simulink model "roadIntersection"  (R2017a)
settings: Solver=VariableStepAuto  StartTime=0  StopTime=40  MaxStep=0.05  RelTol=1e-3
model workspace (MAT data in the model file):
  GREEN_TIME = Simulink.Parameter
  GREEN_TIME.Value = 4
  GREEN_TIME.DataType = 'double'
  GREEN_TIME.Dimensions = [1 1]
  MIN_SAFE_DIST = Simulink.Parameter
  MIN_SAFE_DIST.Value = 1
  MIN_SAFE_DIST.DataType = 'double'
  MIN_SAFE_DIST.Dimensions = [1 1]
  PCROSS_TIME = Simulink.Parameter
  PCROSS_TIME.Value = 3
  PCROSS_TIME.DataType = 'double'
  PCROSS_TIME.Dimensions = [1 1]
  V_MIN = Simulink.Parameter
  V_MIN.Value = 0.25
  V_MIN.DataType = 'double'
  V_MIN.Dimensions = [1 1]
  V_TURN = Simulink.Parameter
  V_TURN.Value = 1.2
  V_TURN.DataType = 'double'
  V_TURN.Dimensions = [1 1]
  WORLD_SIZE = Simulink.Parameter
  WORLD_SIZE.Value = 8
  WORLD_SIZE.DataType = 'double'
  WORLD_SIZE.Dimensions = [1 1]
  YELLOW_TIME = Simulink.Parameter
  YELLOW_TIME.Value = 1
  YELLOW_TIME.DataType = 'double'
  YELLOW_TIME.Dimensions = [1 1]
  dt = Simulink.Parameter
  dt.Value = 0.05
  dt.DataType = 'double'
  dt.DocUnits = 'sec'
  dt.Dimensions = [1 1]
values from neighbouring files (symbols this model uses):
  D = getSimulinkBlockHandle('experiment/Orientation')    [configModel.m]
  m = rt.find('-isa','Simulink.BlockDiagram','-and','Name',mdl)    [configModel.m]
  MIN_SAFE_DIST = 1    [simulation.m]    (also in stateflowSim.m)
  V = getSimulinkBlockHandle('experiment/Velocity')    [configModel.m]
  WORLD_SIZE = 8    [simulation.m]    (also in stateflowSim.m)
  X = getSimulinkBlockHandle('experiment/Position')    [configModel.m]
undefined symbols (not defined in the file or in its folder): DrivingState, n, Stateflow
libraries: libraries x28
(part 1 of 2)
settings Model: Creator=larry  LastModifiedBy=larry
settings SolverCC: ZeroCrossControl=DisableAll  AutoInsertRateTranBlk=on

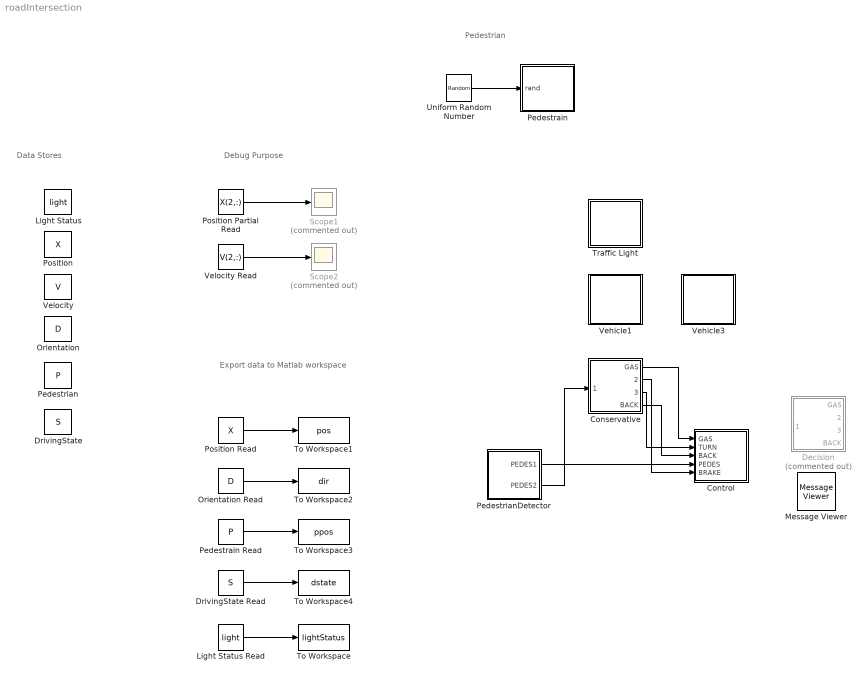
== system roadIntersection ==
  note: Data Stores
  note: Debug Purpose
  note: Export data to
      | Matlab workspace
  note: Pedestrian
  Conservative : Stateflow chart  TreatAsAtomicUnit=on
  Control : Stateflow chart  TreatAsAtomicUnit=on
  Decision : Stateflow chart  Commented=on  TreatAsAtomicUnit=on
  DrivingState : DataStoreMemory  DataStoreName=S  InitialValue=[DrivingState.Straight DrivingState.Straight DrivingState.Straight DrivingState.Straight]  ShowAdditionalParam=off  OutDataTypeStr=Enum: DrivingState
  DrivingState Read : DataStoreRead  DataStoreName=S
  Light Status : DataStoreMemory  DataStoreName=light  ShowAdditionalParam=off  OutDataTypeStr=double  Dimensions=1
  Light Status Read : DataStoreRead  DataStoreName=light
  Message Viewer : MessageViewer
  Orientation : DataStoreMemory  DataStoreName=D  InitialValue=[1 0 -1;0 1 0]  ShowAdditionalParam=off  OutDataTypeStr=double
  Orientation Read : DataStoreRead  DataStoreName=D
  Pedestrain : Stateflow chart  TreatAsAtomicUnit=on
  Pedestrain Read : DataStoreRead  DataStoreName=P
  Pedestrian : DataStoreMemory  DataStoreName=P  InitialValue=[-1; -1; -1; -1]  ShowAdditionalParam=off  OutDataTypeStr=double
  PedestrianDetector : Stateflow chart  TreatAsAtomicUnit=on
  Position : DataStoreMemory  DataStoreName=X  InitialValue=[-6 0.5 6;-0.5 4 0.5]  ShowAdditionalParam=off  OutDataTypeStr=double
  Position Read : DataStoreRead  DataStoreName=X
  Position Partial Read : DataStoreRead  DataStoreName=X  DataStoreElements=X(2,:)
  Scope1 : Scope  Commented=on
  Scope2 : Scope  Commented=on
  To Workspace : ToWorkspace  VariableName=lightStatus  SampleTime=-1
  To Workspace1 : ToWorkspace  VariableName=pos  SampleTime=-1
  To Workspace2 : ToWorkspace  VariableName=dir  SampleTime=-1
  To Workspace3 : ToWorkspace  VariableName=ppos  SampleTime=-1
  To Workspace4 : ToWorkspace  VariableName=dstate  SampleTime=-1
  Traffic Light : Stateflow chart  TreatAsAtomicUnit=on
  Uniform Random Number : UniformRandomNumber  Minimum=0  Maximum=5  SampleTime=0.05
  Vehicle1 : Stateflow chart  TreatAsAtomicUnit=on
  Vehicle3 : Stateflow chart  TreatAsAtomicUnit=on
  Velocity : DataStoreMemory  DataStoreName=V  InitialValue=[0 0 0;0 0 0]  ShowAdditionalParam=off  OutDataTypeStr=double
  Velocity Read : DataStoreRead  DataStoreName=V  DataStoreElements=V(2,:)
  wires:
  Light Status Read/1 -> To Workspace/1
  Position Partial Read/1 -> Scope1/1
  Velocity Read/1 -> Scope2/1
  Position Read/1 -> To Workspace1/1
  Orientation Read/1 -> To Workspace2/1
  Uniform Random Number/1 -> Pedestrain/1(rand)
  Pedestrain Read/1 -> To Workspace3/1
  Conservative/1(GAS) -> Control/1(GAS)
  Conservative/3(TURN) -> Control/2(TURN)
  Conservative/4(BACK) -> Control/3(BACK)
  PedestrianDetector/1(PEDES1) -> Control/4(PEDES)
  Conservative/2(BRAKE) -> Control/5(BRAKE)
  PedestrianDetector/2(PEDES2) -> Conservative/1(PEDES)
  DrivingState Read/1 -> To Workspace4/1

== stateflow chart roadIntersection/Vehicle1 ==
  note: Decision
  note: Perception
  note: Helper
  state Turn
    en:
    completed = false;
    state Right
      en:
      [pf,df] = ...
      prepareRight(this);
      ex:
      inter = resumeFromRight(this, df);
      state Turn
      state TurnStop
      (default) -> Turn.Right.Turn
      Turn.Right.TurnStop -> Turn.Right.Turn : [~hasPedestrian(this)]
      Turn.Right.Turn -> Turn.Right.TurnStop : [hasPedestrian(this)]
    state Left
      en:
      [pf, df] = ...
      prepareLeft(this);
      ex:
      inter = resumeFromLeft(this, df);
      state Turn
      state TurnStop
      (default) -> Turn.Left.Turn
      Turn.Left.TurnStop -> Turn.Left.Turn : [~hasPedestrian(this)]
      Turn.Left.Turn -> Turn.Left.TurnStop : [hasPedestrian(this)]
    (default) -> Right [order 1] : [decision == Decision.Right]
    (default) -> Left [order 2]
  state GoStraight
    state FreeDriving
    state Follow
      en:
      front = frontCarIndex(this);
      state FollowBehind
    (default) -> GoStraight.FreeDriving [order 2]
    GoStraight.FreeDriving -> GoStraight.Follow : [hasFrontCar(this)]
    GoStraight.Follow -> GoStraight.FreeDriving : [frontCarHasLeft(this)]
    (default) -> GoStraight.Follow [order 1] : [hasFrontCar(this)]
  state RoadIntersection
    state Normal
      state FreeDriving
        state AccToHighestRate
        state SlowDownToStop
        state SlowAdjust
        state RushToPass
        (default) -> (junction 88) [order 2]
        (default) -> AccToHighestRate [order 1] : [isGreen(this)]
        AccToHighestRate -> (junction 88) : [isYellow(this)]
        (junction 88) -> (junction 177) [order 2]
        (junction 88) -> RoadIntersection.Normal.FreeDriving.SlowAdjust [order 1] : [isStopped(this)]...
            | {obj = inter;}
        RoadIntersection.Normal.FreeDriving.SlowAdjust -> AccToHighestRate : [isGreen(this)]
        SlowDownToStop -> AccToHighestRate : [isGreen(this)]
        (junction 177) -> SlowDownToStop [order 1] : [isStoppable(this,inter)]...
            | {a_norm = requiredBrake(...
            | this,inter);}
        (junction 177) -> RushToPass [order 2]
      state Follow
        en:
        front = frontCarIndex(this);
        obj = X(:,front);
        du:
        obj = closestObj(this, obj, inter);
        state FollowBehind
        state NonStopFollow
        state SlowAdjust
        (default) -> (junction 164) [order 2]
        (default) -> RoadIntersection.Normal.Follow.FollowBehind [order 1] : [isGreen(this)]
        RoadIntersection.Normal.Follow.FollowBehind -> (junction 164) : [isYellow(this)]
        (junction 164) -> RoadIntersection.Normal.Follow.SlowAdjust [order 1] : [isStoppable(this,obj)]
        (junction 164) -> NonStopFollow [order 2]
        RoadIntersection.Normal.Follow.SlowAdjust -> RoadIntersection.Normal.Follow.FollowBehind : [isGreen(this)]
      (default) -> RoadIntersection.Normal.FreeDriving [order 2]
      (default) -> RoadIntersection.Normal.Follow [order 1] : [hasFrontCar(this)]
      RoadIntersection.Normal.FreeDriving -> RoadIntersection.Normal.Follow : [hasFrontCar(this)]
      RoadIntersection.Normal.Follow -> RoadIntersection.Normal.FreeDriving : [frontCarHasLeft(this)]
    state Pedestrian
      state EmergenceStop
    (default) -> Normal [order 2]
    Normal -> Pedestrian : [hasPedestrian(this)]
    Pedestrian -> Normal : [~hasPedestrian(this)]
    (default) -> Pedestrian [order 1] : [hasPedestrian(this)]
  (default) -> GoStraight
  Turn -> GoStraight : [completed]
  (junction 195) -> GoStraight [order 1] : [decision == Decision.Straight]
  GoStraight -> RoadIntersection : [isCloseTo(this,inter)]
  (junction 195) -> Turn [order 2]
  RoadIntersection -> (junction 195) : [passStopLine(this)]
  data: this function_input; completed function_output; d2 function_input; p2 function_input; this function_input; p2 function_input; this function_input; completed function_output; d2 function_input; p2 function_input; this function_input; p2 function_input; v_target function_input; a_norm function_input; this function_input; a_max function_input; this function_input; front function_input; self function_input; res function_output; self function_input; obj1 function_input; res function_output; obj2 function_input; self function_input; pos function_input; res function_output; self function_input; res function_output; self function_input; idx function_output; self function_input uint8 size=1; d function_input; newInnter function_output; self function_input; res function_output; pos function_input; self function_input; pos function_input; res function_output; self function_input uint8 size=1; p function_output; d function_output; self function_input; res function_output; self function_input uint8 size=1; d function_input; newInter function_output; self function_input uint8 size=1; p function_output; d function_output; self function_input; res function_output; self function_input; res function_output; self function_input; res function_output; v_target function_input; a_norm function_input; this function_input; a_norm function_input; this function_input; this function_input; a_norm function_input; obj function_input; v_target function_input; a_norm function_input; this function_input; a_max function_input; this function_input; front function_input; a_max function_input; this function_input; front function_input; this function_input; a_norm function_input; obj function_input; a_norm function_input; this function_input; self function_input uint8 size=1; res function_output boolean size=1; dt parameter double size=1; this local uint8 =uint8(1); V data_store_memory; X data_store_memory size=[1 2]; D data_store_memory; A_MAX local double =2.5; V_MAX local double =2.5; light data_store_memory; inter local double size=[2 1] =[-1; -0.5]; MIN_SAFE_DIST parameter; a_norm local double size=1 =0; WORLD_SIZE parameter; front local uint8 size=1; obj local double size=[2 1]; V_MIN parameter; decision local Enum: Decision size=1 =Decision.Straight; completed local boolean size=1 =false; P data_store_memory; df local double size=[2 1]; pf local double size=[2 1]
  function res = hasPedestrian(self):
    | function res = hasPedestrian(self)
    | 
    | if ~any(P ~= -1)
    |     res = false;
    |     return;
    | end
    | 
    | FARAWAY = 100;
    | 
    | pi = [-1 1 1 -1; -1 -1 1 1];
    | dp = [2 0 -2 0; 0 2 0 -2];
    | 
    | dx_norm = ones(4, 1) * FARAWAY;
    | x = X(:,self);
    | d = D(:,self);
    | 
    | for k=1:length(P)
    |     if P(k) ~= -1
    |         p = pi(:,k) + dp(:,k) * P(k); 
    |         dx = p - x;
    |         check = dot(dx, d);
    |         if check > 0
    |             dx_norm(k) = norm(dx);
    |             theta = acos(check/dx_norm(k));
    |             if rad2deg(theta) > 10
    |                 dx_norm(k) = FARAWAY;
    |             end
    |         end
    |     end
    | end
    | 
    | res = any(dx_norm <= 1 * MIN_SAFE_DIST);
  function res = closestObj(self, obj1, obj2):
    | function res = closestObj(self, obj1, obj2)
    | 
    | if isequal(obj1, obj2)
    |     res = obj1;
    |     return;
    | end
    | 
    | RANGE = 2*WORLD_SIZE;
    | 
    | x = X(:,self);
    | d = D(:,self);
    | 
    | dX = zeros(2, 1);
    | dX(1) = mod(dot(obj1 - x, d) + RANGE, RANGE);
    | dX(2) = mod(dot(obj2 - x, d) + RANGE, RANGE);
    | 
    | [~, index] = min(dX);
    | if index == 1
    |     res = obj1;
    | else
    |     res = obj2;
    | end
  function res = isStoppable(self,pos):
    | function res = isStoppable(self,pos)
    | 
    | x = X(:,self);
    | v = V(:,self);
    | d = D(:,self);
    | 
    | range = 2 * WORLD_SIZE;
    | diff = mod((dot(pos - x, d)+range), range) ;
    | dist = diff - MIN_SAFE_DIST;
    | 
    | v_norm = norm(v);
    | brake_dist = v_norm*v_norm/2.0/A_MAX;
    | res = (brake_dist <= dist);
  function res = passStopLine(self):
    | function res = passStopLine(self)
    | 
    | x = X(:,self);
    | d = D(:,self);
    | 
    | dx_norm = dot(inter - x, d);
    | res = (dx_norm <= 0);
  function idx = frontCarIndex(self):
    | function idx = frontCarIndex(self)
    | 
    | FARAWAY = 100;
    | RANGE = 2*WORLD_SIZE;
    | 
    | dx = zeros(size(X, 2), 1);
    | x = X(:,self);
    | v = V(:,self);
    | d = D(:,self);
    | 
    | for k=1:length(dx)
    |     dx(k) = dot(X(:,k) - x, d);
    |     dx(k) = mod((dx(k)+RANGE), RANGE);
    | end
    | 
    | % set zero dX to a large enough value
    | dx(dx == 0) = FARAWAY;
    | [~, idx] = min(dx);
    | idx = uint8(idx);
  function newInnter = resumeFromRight(self, d):
    | function newInnter = resumeFromRight(self, d)
    | 
    | x = X(:,self);
    | 
    | if isequal(d, [0; -1])
    |     x = [-0.5; -1];
    |     newInnter = [-0.5; 1];
    | elseif isequal(d, [0; 1])
    |     x = [0.5; 1];
    |     newInnter = [-0.5; -1];
    | elseif isequal(d, [1; 0])
    |     x = [1; -0.5];
    |     newInnter = [-1; -0.5];
    | elseif isequal(d, [-1; 0])
    |     x = [-1; 0.5];
    |     newInnter = [1; 0.5];
    | else
    |     error('Unknown orientation');
    | end
    | 
    | v = V(:,self);
    | 
    | X(:,self) = x;
    | V(:,self) = d * norm(v);
    | D(:,self) = d;
  function res = isCloseTo(self,pos):
    | function res = isCloseTo(self,pos)
    | 
    | x = X(:,self);
    | d = D(:,self);
    | 
    | dist = dot(pos-x, d);
    | res = ((dist > 0) && (dist <= 2.5*MIN_SAFE_DIST));
  function res = requiredBrake(self,pos):
    | function res = requiredBrake(self,pos)
    | 
    | x = X(:,self);
    | v = V(:,self);
    | d = D(:,self);
    | 
    | % add safe distance
    | range = 2 * WORLD_SIZE;
    | diff = mod((dot(pos - x, d)+range),range);
    | dist = diff - MIN_SAFE_DIST;
    | % assert(dist >= 0, 'Error in required Brake');
    | 
    | vnorm = norm(v);
    | res = vnorm*vnorm/2/dist;
  function [p, d] = prepareRight(self):
    | function [p, d] = prepareRight(self)
    | 
    | d0 = D(:,self);
    | p = [0; 0];
    | d = [0; 0];
    | 
    | if isequal(d0, [1; 0])
    |     p = [-0.5; -1];
    |     d = [0; -1];
    | elseif isequal(d0, [-1; 0])
    |     p = [0.5; 1];
    |     d = [0; 1];
    | elseif isequal(d0, [0; 1])
    |     p = [1; -0.5];
    |     d = [1; 0];
    | elseif isequal(d0, [0; -1])
    |     p = [-1; 0.5];
    |     d = [-1; 0];
    | else
    |     error('Unknown orientation');
    | end
  function res = isGreen(self):
    | function res = isGreen(self)
    | 
    | d = D(:,self);
    | 
    | % compute the corresponding traffic light
    | horizon = (abs(d(1)) ~= 0);
    | vertical = (abs(d(2)) ~= 0);
    | 
    | res = false;
    | if uint8(light) == 3 && horizon
    |     % horizontal: green, vertical: red
    |     res = true;
    | elseif uint8(light) == 1 && vertical
    |     % horizontal: red, vertical: green
    |     res = true;
    | end
  function newInter = resumeFromLeft(self, d):
    | function newInter = resumeFromLeft(self, d)
    | 
    | x = X(:,self);
    | v = V(:,self);
    | 
    | if isequal(d, [1; 0])
    |     x = [1; -0.5];
    |     newInter = [-1; -0.5];
    | elseif isequal(d, [-1; 0])
    |     x = [-1; 0.5];
    |     newInter = [1; 0.5];
    | elseif isequal(d, [0; 1])
    |     x = [0.5; 1];
    |     newInter = [0.5; -1];
    | elseif isequal(d, [0; -1])
    |     x = [-0.5; -1];
    |     newInter = [-0.5; 1];
    | else
    |     error('Unknown orientation');
    | end
    | 
    | X(:,self) = x;
    | V(:,self) = d * norm(v);
    | D(:,self) = d;
  function [p, d] = prepareLeft(self):
    | function [p, d] = prepareLeft(self)
    | 
    | d0 = D(:,self);
    | p = [0; 0];
    | d = [0; 0];
    | 
    | if isequal(d0, [1; 0])
    |     p = [0.5; 1];
    |     d = [0; 1];
    | elseif isequal(d0, [-1; 0])
    |     p = [-0.5; -1];
    |     d = [0; -1];
    | elseif isequal(d0, [0; 1])
    |     p = [-1; 0.5];
    |     d = [-1; 0];
    | elseif isequal(d0, [0; -1])
    |     p = [1; -0.5];
    |     d = [1; 0];
    | else
    |     error('Unknown orientation');
    | end
  function res = isYellow(self):
    | function res = isYellow(self)
    | 
    | d = D(:,self);
    | 
    | % compute the corresponding traffic light
    | horizon = (abs(d(1)) ~= 0);
    | vertical = (abs(d(2)) ~= 0);
    | 
    | res = false;
    | if uint8(light) == 4 && horizon
    |     % horizontal: yellow, vertical: red
    |     res = true;
    | elseif uint8(light) == 2 && vertical
    |     % horizontal: red, vertical: yellow
    |     res = true;
    | end
  function res = hasFrontCar(self):
    | function res = hasFrontCar(self)
    | 
    | % constants
    | THRES = 2 * MIN_SAFE_DIST;
    | FARAWAY = 100;
    | RANGE = 2 * WORLD_SIZE;
    | 
    | res = false;
    | 
    | % row of X: coordinate, col of X: num of cars
    | num = size(X, 2);
    | if num == 1
    |     return;
    | end
    | 
    | dx = zeros(num, 1);
    | x = X(:,self);
    | d = D(:,self);
    | car_size = [0.3; 0.4];
    | 
    | for k=1:length(dx)
    |     
    |     % compute difference
    |     xdelta = X(:,k) - x;
    |     
    |     % parallel and vertical distance
    |     delta_p = dot(xdelta, d);
    |     delta_v = norm(xdelta - (d * delta_p));
    |     
    |     % vertical distance is larger than car width
    |     if delta_v < car_size(1)
    |         dx(k) = delta_p;
    |     else
    |         dx(k) = FARAWAY;
    |     end
    |     
    |     % a rounded world
    |     dx(k) = mod((dx(k)+RANGE), RANGE);
    | end
    | 
    | % set zero dX to a large enough value
    | dx(dx == 0) = FARAWAY;
    | closest = min(dx);
    | res = closest <= THRES;
  function res = frontCarHasLeft(self):
    | function res = frontCarHasLeft(self)
    | 
    | % Constants 
    | THRES = 2.5 * MIN_SAFE_DIST;
    | FARAWAY = 100;
    | RANGE = 2 * WORLD_SIZE;
    | 
    | % if only one car in the environment return directly
    | res = true;
    | num = size(X, 1);
    | if num == 1
    |     return;
    | end
    | 
    | % get the closet car index and its distance
    | dx = zeros(num, 1);
    | x = X(:,self);
    | d = D(:,self);
    | car_size = [0.3; 0.4];
    | 
    | for k=1:length(dx)
    |     
    |     xdelta = X(:,k) - x;
    |     xdelta_p = dot(xdelta, d);                  % parallel component
    |     xdelta_v = norm(xdelta - (d * xdelta_p));   % vertical component
    |     
    |     % when the vertical component is larger than the car width
    |     if xdelta_v < car_size(1)
    |         dx(k) = xdelta_p;
    |     else
    |         dx(k) = FARAWAY;
    |     end
    |     
    |     % since we are in the round world, normalize the distance if the 
    |     % front car is behind us 
    |     % a rounded world
    |     dx(k) = mod((dx(k)+RANGE), RANGE);
    | end
    | 
    | % set the zero dx to a large enough value for convenience
    | dx(dx == 0) = FARAWAY;
    | closest = min(dx);
    | res = closest > THRES;
  function res = isStopped(self):
    | function res = isStopped(self)
    | 
    | v = V(:,self);
    | d = D(:,self);
    | res = (dot(v, d) <= 0)||(norm(v) < V_MIN);

== stateflow chart roadIntersection/Vehicle3 ==
  note: Decision
  note: Perception
  note: Helper
  state Turn
    en:
    completed = false;
    state Right
      en:
      [pf,df] = ...
      prepareRight(this);
      ex:
      inter = resumeFromRight(this, df);
      state Turn
      state TurnStop
      (default) -> Turn.Right.Turn
      Turn.Right.TurnStop -> Turn.Right.Turn : [~hasPedestrian(this)]
      Turn.Right.Turn -> Turn.Right.TurnStop : [hasPedestrian(this)]
    state Left
      en:
      [pf, df] = ...
      prepareLeft(this);
      ex:
      inter = resumeFromLeft(this, df);
      state Turn
      state TurnStop
      (default) -> Turn.Left.Turn
      Turn.Left.TurnStop -> Turn.Left.Turn : [~hasPedestrian(this)]
      Turn.Left.Turn -> Turn.Left.TurnStop : [hasPedestrian(this)]
    (default) -> Right [order 1] : [decision == Decision.Right]
    (default) -> Left [order 2]
  state GoStraight
    state FreeDriving
    state Follow
      en:
      front = frontCarIndex(this);
      state FollowBehind
    (default) -> GoStraight.FreeDriving [order 2]
    GoStraight.FreeDriving -> GoStraight.Follow : [hasFrontCar(this)]
    GoStraight.Follow -> GoStraight.FreeDriving : [frontCarHasLeft(this)]
    (default) -> GoStraight.Follow [order 1] : [hasFrontCar(this)]
  state RoadIntersection
    state Normal
      state FreeDriving
        state AccToHighestRate
        state SlowDownToStop
        state SlowAdjust
        state RushToPass
        (default) -> (junction 88) [order 2]
        (default) -> AccToHighestRate [order 1] : [isGreen(this)]
        AccToHighestRate -> (junction 88) : [isYellow(this)]
        (junction 88) -> (junction 177) [order 2]
        (junction 88) -> RoadIntersection.Normal.FreeDriving.SlowAdjust [order 1] : [isStopped(this)]...
            | {obj = inter;}
        RoadIntersection.Normal.FreeDriving.SlowAdjust -> AccToHighestRate : [isGreen(this)]
        SlowDownToStop -> AccToHighestRate : [isGreen(this)]
        (junction 177) -> SlowDownToStop [order 1] : [isStoppable(this,inter)]...
            | {a_norm = requiredBrake(...
            | this,inter);}
        (junction 177) -> RushToPass [order 2]
      state Follow
        en:
        front = frontCarIndex(this);
        obj = X(:,front);
        du:
        obj = closestObj(this, obj, inter);
        state FollowBehind
        state NonStopFollow
        state SlowAdjust
        (default) -> (junction 164) [order 2]
        (default) -> RoadIntersection.Normal.Follow.FollowBehind [order 1] : [isGreen(this)]
        RoadIntersection.Normal.Follow.FollowBehind -> (junction 164) : [isYellow(this)]
        (junction 164) -> RoadIntersection.Normal.Follow.SlowAdjust [order 1] : [isStoppable(this,obj)]
        (junction 164) -> NonStopFollow [order 2]
        RoadIntersection.Normal.Follow.SlowAdjust -> RoadIntersection.Normal.Follow.FollowBehind : [isGreen(this)]
      (default) -> RoadIntersection.Normal.FreeDriving [order 2]
      (default) -> RoadIntersection.Normal.Follow [order 1] : [hasFrontCar(this)]
      RoadIntersection.Normal.FreeDriving -> RoadIntersection.Normal.Follow : [hasFrontCar(this)]
      RoadIntersection.Normal.Follow -> RoadIntersection.Normal.FreeDriving : [frontCarHasLeft(this)]
    state Pedestrian
      state EmergenceStop
    (default) -> Normal [order 2]
    Normal -> Pedestrian : [hasPedestrian(this)]
    Pedestrian -> Normal : [~hasPedestrian(this)]
    (default) -> Pedestrian [order 1] : [hasPedestrian(this)]
  (default) -> GoStraight
  Turn -> GoStraight : [completed]
  (junction 195) -> GoStraight [order 1] : [decision == Decision.Straight]
  GoStraight -> RoadIntersection : [isCloseTo(this,inter)]
  (junction 195) -> Turn [order 2]
  RoadIntersection -> (junction 195) : [passStopLine(this)]
  data: this function_input; completed function_output; d2 function_input; p2 function_input; this function_input; p2 function_input; this function_input; completed function_output; d2 function_input; p2 function_input; this function_input; p2 function_input; v_target function_input; a_norm function_input; this function_input; a_max function_input; this function_input; front function_input; self function_input; res function_output; self function_input; obj1 function_input; res function_output; obj2 function_input; self function_input; pos function_input; res function_output; self function_input; res function_output; self function_input; idx function_output; self function_input uint8 size=1; d function_input; newInnter function_output; self function_input; res function_output; pos function_input; self function_input; pos function_input; res function_output; self function_input uint8 size=1; p function_output; d function_output; self function_input; res function_output; self function_input uint8 size=1; d function_input; newInter function_output; self function_input uint8 size=1; p function_output; d function_output; self function_input; res function_output; self function_input; res function_output; self function_input; res function_output; v_target function_input; a_norm function_input; this function_input; a_norm function_input; this function_input; this function_input; a_norm function_input; obj function_input; v_target function_input; a_norm function_input; this function_input; a_max function_input; this function_input; front function_input; a_max function_input; this function_input; front function_input; this function_input; a_norm function_input; obj function_input; a_norm function_input; this function_input; self function_input uint8 size=1; res function_output boolean size=1; dt parameter double size=1; this local uint8 =uint8(3); V data_store_memory; X data_store_memory size=[1 2]; D data_store_memory; A_MAX local double =2.5; V_MAX local double =2.5; light data_store_memory; inter local double size=[2 1] =[1; 0.5]; MIN_SAFE_DIST parameter; a_norm local double size=1 =0; WORLD_SIZE parameter; front local uint8 size=1; obj local double size=[2 1]; V_MIN parameter; decision local Enum: Decision size=1 =Decision.Straight; completed local boolean size=1 =false; P data_store_memory; df local double size=[2 1]; pf local double size=[2 1]
  function res = hasPedestrian(self):
    | function res = hasPedestrian(self)
    | 
    | if ~any(P ~= -1)
    |     res = false;
    |     return;
    | end
    | 
    | FARAWAY = 100;
    | 
    | pi = [-1 1 1 -1; -1 -1 1 1];
    | dp = [2 0 -2 0; 0 2 0 -2];
    | 
    | dx_norm = ones(4, 1) * FARAWAY;
    | x = X(:,self);
    | d = D(:,self);
    | 
    | for k=1:length(P)
    |     if P(k) ~= -1
    |         p = pi(:,k) + dp(:,k) * P(k); 
    |         dx = p - x;
    |         check = dot(dx, d);
    |         if check > 0
    |             dx_norm(k) = norm(dx);
    |             theta = acos(check/dx_norm(k));
    |             if rad2deg(theta) > 10
    |                 dx_norm(k) = FARAWAY;
    |             end
    |         end
    |     end
    | end
    | 
    | res = any(dx_norm <= 1 * MIN_SAFE_DIST);
  function res = closestObj(self, obj1, obj2):
    | function res = closestObj(self, obj1, obj2)
    | 
    | if isequal(obj1, obj2)
    |     res = obj1;
    |     return;
    | end
    | 
    | RANGE = 2*WORLD_SIZE;
    | 
    | x = X(:,self);
    | d = D(:,self);
    | 
    | dX = zeros(2, 1);
    | dX(1) = mod(dot(obj1 - x, d) + RANGE, RANGE);
    | dX(2) = mod(dot(obj2 - x, d) + RANGE, RANGE);
    | 
    | [~, index] = min(dX);
    | if index == 1
    |     res = obj1;
    | else
    |     res = obj2;
    | end
  function res = isStoppable(self,pos):
    | function res = isStoppable(self,pos)
    | 
    | x = X(:,self);
    | v = V(:,self);
    | d = D(:,self);
    | 
    | range = 2 * WORLD_SIZE;
    | diff = mod((dot(pos - x, d)+range), range) ;
    | dist = diff - MIN_SAFE_DIST;
    | 
    | v_norm = norm(v);
    | brake_dist = v_norm*v_norm/2.0/A_MAX;
    | res = (brake_dist <= dist);
  function res = passStopLine(self):
    | function res = passStopLine(self)
    | 
    | x = X(:,self);
    | d = D(:,self);
    | 
    | dx_norm = dot(inter - x, d);
    | res = (dx_norm <= 0);
  function idx = frontCarIndex(self):
    | function idx = frontCarIndex(self)
    | 
    | FARAWAY = 100;
    | RANGE = 2*WORLD_SIZE;
    | 
    | dx = zeros(size(X, 2), 1);
    | x = X(:,self);
    | v = V(:,self);
    | d = D(:,self);
    | 
    | for k=1:length(dx)
    |     dx(k) = dot(X(:,k) - x, d);
    |     dx(k) = mod((dx(k)+RANGE), RANGE);
    | end
    | 
    | % set zero dX to a large enough value
    | dx(dx == 0) = FARAWAY;
    | [~, idx] = min(dx);
    | idx = uint8(idx);
  function newInnter = resumeFromRight(self, d):
    | function newInnter = resumeFromRight(self, d)
    | 
    | x = X(:,self);
    | 
    | if isequal(d, [0; -1])
    |     x = [-0.5; -1];
    |     newInnter = [-0.5; 1];
    | elseif isequal(d, [0; 1])
    |     x = [0.5; 1];
    |     newInnter = [-0.5; -1];
    | elseif isequal(d, [1; 0])
    |     x = [1; -0.5];
    |     newInnter = [-1; -0.5];
    | elseif isequal(d, [-1; 0])
    |     x = [-1; 0.5];
    |     newInnter = [1; 0.5];
    | else
    |     error('Unknown orientation');
    | end
    | 
    | v = V(:,self);
    | 
    | X(:,self) = x;
    | V(:,self) = d * norm(v);
    | D(:,self) = d;
  function res = isCloseTo(self,pos):
    | function res = isCloseTo(self,pos)
    | 
    | x = X(:,self);
    | d = D(:,self);
    | 
    | dist = dot(pos-x, d);
    | res = ((dist > 0) && (dist <= 2.5*MIN_SAFE_DIST));
  function res = requiredBrake(self,pos):
    | function res = requiredBrake(self,pos)
    | 
    | x = X(:,self);
    | v = V(:,self);
    | d = D(:,self);
    | 
    | % add safe distance
    | range = 2 * WORLD_SIZE;
    | diff = mod((dot(pos - x, d)+range),range);
    | dist = diff - MIN_SAFE_DIST;
    | % assert(dist >= 0, 'Error in required Brake');
    | 
    | vnorm = norm(v);
    | res = vnorm*vnorm/2/dist;
  function [p, d] = prepareRight(self):
    | function [p, d] = prepareRight(self)
    | 
    | d0 = D(:,self);
    | p = [0; 0];
    | d = [0; 0];
    | 
    | if isequal(d0, [1; 0])
    |     p = [-0.5; -1];
    |     d = [0; -1];
    | elseif isequal(d0, [-1; 0])
    |     p = [0.5; 1];
    |     d = [0; 1];
    | elseif isequal(d0, [0; 1])
    |     p = [1; -0.5];
    |     d = [1; 0];
    | elseif isequal(d0, [0; -1])
    |     p = [-1; 0.5];
    |     d = [-1; 0];
    | else
    |     error('Unknown orientation');
    | end
  function res = isGreen(self):
    | function res = isGreen(self)
    | 
    | d = D(:,self);
    | 
    | % compute the corresponding traffic light
    | horizon = (abs(d(1)) ~= 0);
    | vertical = (abs(d(2)) ~= 0);
    | 
    | res = false;
    | if uint8(light) == 3 && horizon
    |     % horizontal: green, vertical: red
    |     res = true;
    | elseif uint8(light) == 1 && vertical
    |     % horizontal: red, vertical: green
    |     res = true;
    | end
  function newInter = resumeFromLeft(self, d):
    | function newInter = resumeFromLeft(self, d)
    | 
    | x = X(:,self);
    | v = V(:,self);
    | 
    | if isequal(d, [1; 0])
    |     x = [1; -0.5];
    |     newInter = [-1; -0.5];
    | elseif isequal(d, [-1; 0])
    |     x = [-1; 0.5];
    |     newInter = [1; 0.5];
    | elseif isequal(d, [0; 1])
    |     x = [0.5; 1];
    |     newInter = [0.5; -1];
    | elseif isequal(d, [0; -1])
    |     x = [-0.5; -1];
    |     newInter = [-0.5; 1];
    | else
    |     error('Unknown orientation');
    | end
    | 
    | X(:,self) = x;
    | V(:,self) = d * norm(v);
    | D(:,self) = d;
  function [p, d] = prepareLeft(self):
    | function [p, d] = prepareLeft(self)
    | 
    | d0 = D(:,self);
    | p = [0; 0];
    | d = [0; 0];
    | 
    | if isequal(d0, [1; 0])
    |     p = [0.5; 1];
    |     d = [0; 1];
    | elseif isequal(d0, [-1; 0])
    |     p = [-0.5; -1];
    |     d = [0; -1];
    | elseif isequal(d0, [0; 1])
    |     p = [-1; 0.5];
    |     d = [-1; 0];
    | elseif isequal(d0, [0; -1])
    |     p = [1; -0.5];
    |     d = [1; 0];
    | else
    |     error('Unknown orientation');
    | end
  function res = isYellow(self):
    | function res = isYellow(self)
    | 
    | d = D(:,self);
    | 
    | % compute the corresponding traffic light
    | horizon = (abs(d(1)) ~= 0);
    | vertical = (abs(d(2)) ~= 0);
    | 
    | res = false;
    | if uint8(light) == 4 && horizon
    |     % horizontal: yellow, vertical: red
    |     res = true;
    | elseif uint8(light) == 2 && vertical
    |     % horizontal: red, vertical: yellow
    |     res = true;
    | end
  function res = hasFrontCar(self):
    | function res = hasFrontCar(self)
    | 
    | % constants
    | THRES = 2 * MIN_SAFE_DIST;
    | FARAWAY = 100;
    | RANGE = 2 * WORLD_SIZE;
    | 
    | res = false;
    | 
    | % row of X: coordinate, col of X: num of cars
    | num = size(X, 2);
    | if num == 1
    |     return;
    | end
    | 
    | dx = zeros(num, 1);
    | x = X(:,self);
    | d = D(:,self);
    | car_size = [0.3; 0.4];
    | 
    | for k=1:length(dx)
    |     
    |     % compute difference
    |     xdelta = X(:,k) - x;
    |     
    |     % parallel and vertical distance
    |     delta_p = dot(xdelta, d);
    |     delta_v = norm(xdelta - (d * delta_p));
    |     
    |     % vertical distance is larger than car width
    |     if delta_v < car_size(1)
    |         dx(k) = delta_p;
    |     else
    |         dx(k) = FARAWAY;
    |     end
    |     
    |     % a rounded world
    |     dx(k) = mod((dx(k)+RANGE), RANGE);
    | end
    | 
    | % set zero dX to a large enough value
    | dx(dx == 0) = FARAWAY;
    | closest = min(dx);
    | res = closest <= THRES;
  function res = frontCarHasLeft(self):
    | function res = frontCarHasLeft(self)
    | 
    | % Constants 
    | THRES = 2.5 * MIN_SAFE_DIST;
    | FARAWAY = 100;
    | RANGE = 2 * WORLD_SIZE;
    | 
    | % if only one car in the environment return directly
    | res = true;
    | num = size(X, 1);
    | if num == 1
    |     return;
    | end
    | 
    | % get the closet car index and its distance
    | dx = zeros(num, 1);
    | x = X(:,self);
    | d = D(:,self);
    | car_size = [0.3; 0.4];
    | 
    | for k=1:length(dx)
    |     
    |     xdelta = X(:,k) - x;
    |     xdelta_p = dot(xdelta, d);                  % parallel component
    |     xdelta_v = norm(xdelta - (d * xdelta_p));   % vertical component
    |     
    |     % when the vertical component is larger than the car width
    |     if xdelta_v < car_size(1)
    |         dx(k) = xdelta_p;
    |     else
    |         dx(k) = FARAWAY;
    |     end
    |     
    |     % since we are in the round world, normalize the distance if the 
    |     % front car is behind us 
    |     % a rounded world
    |     dx(k) = mod((dx(k)+RANGE), RANGE);
    | end
    | 
    | % set the zero dx to a large enough value for convenience
    | dx(dx == 0) = FARAWAY;
    | closest = min(dx);
    | res = closest > THRES;
  function res = isStopped(self):
    | function res = isStopped(self)
    | 
    | v = V(:,self);
    | d = D(:,self);
    | res = (dot(v, d) <= 0)||(norm(v) < V_MIN);

== stateflow chart roadIntersection/Traffic Light ==
  state Y_R
    en:
    light = 4;
  state R_G
    en:
    light = 1;
    state Pass
    state NotPass
    (default) -> R_G.Pass
    R_G.Pass -> R_G.NotPass : after(G_TIME-CROSS_TIME,sec)
  state G_R
    en:
    light = 3;
    state Pass
    state NotPass
    (default) -> G_R.Pass
    G_R.Pass -> G_R.NotPass : after(G_TIME-CROSS_TIME,sec)
  state R_Y
    en:
    light = 2;
  Y_R -> R_G : after(Y_TIME, sec)
  G_R -> Y_R : after(G_TIME, sec)
  (default) -> R_G
  R_G -> R_Y : after(G_TIME, sec)
  R_Y -> G_R : after(Y_TIME, sec)
  data: light data_store_memory; CROSS_TIME constant double =3; G_TIME constant double =4; Y_TIME constant double =1

== stateflow chart roadIntersection/Pedestrain ==
  state P_LeftBottom [parallel]
    settings: executionOrder=1
    state Walking
      en:
      P(this) = 0;
      du:
      P(this) = ...
      temporalCount(sec)/PCROSS_TIME;
      ex:
      P(this) = 1;
    state Finish
      en:
      P(this) = -1;
    state Wait
    P_LeftBottom.Walking -> P_LeftBottom.Finish : after(PCROSS_TIME, sec)
    P_LeftBottom.Wait -> P_LeftBottom.Walking : [light == 3]
    P_LeftBottom.Finish -> P_LeftBottom.Wait : [uint8(rand) == this]
    (default) -> P_LeftBottom.Finish
  state P_RightBottom [parallel]
    settings: executionOrder=2
    state Walking
      en:
      P(this) = 0;
      du:
      P(this) = ...
      temporalCount(sec)/PCROSS_TIME;
      ex:
      P(this) = 1;
    state Finish
      en:
      P(this) = -1;
    state Wait
    P_RightBottom.Walking -> P_RightBottom.Finish : after(PCROSS_TIME, sec)
    P_RightBottom.Wait -> P_RightBottom.Walking : [light == 1]
    P_RightBottom.Finish -> P_RightBottom.Wait : [uint8(rand) == this]
    (default) -> P_RightBottom.Finish
  state P_RightTop [parallel]
    settings: executionOrder=3
    state Walking
      en:
      P(this) = 0;
      du:
      P(this) = ...
      temporalCount(sec)/PCROSS_TIME;
      ex:
      P(this) = 1;
    state Finish
      en:
      P(this) = -1;
    state Wait
    P_RightTop.Walking -> P_RightTop.Finish : after(PCROSS_TIME, sec)
    P_RightTop.Wait -> P_RightTop.Walking : [light == 3]
    P_RightTop.Finish -> P_RightTop.Wait : [uint8(rand) == this]
    (default) -> P_RightTop.Finish
  state P_LeftTop [parallel]
    settings: executionOrder=4
    state Walking
      en:
      P(this) = 0;
      du:
      P(this) = ...
      temporalCount(sec)/PCROSS_TIME;
      ex:
      P(this) = 1;
    state Finish
      en:
      P(this) = -1;
    state Wait
    P_LeftTop.Walking -> P_LeftTop.Finish : after(PCROSS_TIME, sec)
    P_LeftTop.Wait -> P_LeftTop.Walking : [light == 1]
    P_LeftTop.Finish -> P_LeftTop.Wait : [uint8(rand) == this]
    (default) -> P_LeftTop.Finish
  data: this local uint8 size=1 =uint8(1); this local uint8 size=1 =uint8(2); this local uint8 size=1 =uint8(3); this local uint8 size=1 =uint8(4); light data_store_memory; PCROSS_TIME parameter; P data_store_memory; rand input

== stateflow chart roadIntersection/Control ==
  state res = receiveBack [function]
    (default) -> (junction 120) : {res = false;}
    (junction 120) -> (junction 113) [order 1] : BACK
    (junction 113) -> (junction 115) : {TRASH.data = zeros(2,1);
        | forward(BACK,TRASH);}
    (junction 115) -> (junction 120) : {res = true;}
    (junction 120) -> (junction 116) [order 2]
  state res = receiveTurn [function]
    (default) -> (junction 102) : {msgData = zeros(0,1);
        | res = false;}
    (junction 102) -> (junction 106) [order 1] : TURN
    (junction 106) -> (junction 107) : {msgData = TURN.data;
        | TRASH.data = TURN.data;
        | forward(TURN,TRASH);}
    (junction 107) -> (junction 102) : {res = true;}
    (junction 102) -> (junction 110) [order 2]
  state res = receiveGas [function]
    (default) -> (junction 87) : {msgData = zeros(0,1);
        | res = false;}
    (junction 87) -> (junction 86) [order 1] : GAS
    (junction 86) -> (junction 88) : {msgData = GAS.data;
        | TRASH.data = GAS.data;
        | forward(GAS,TRASH);}
    (junction 88) -> (junction 87) : {res = true;}
    (junction 87) -> (junction 89) [order 2]
  state res = needSlowDown [function]
    (default) -> (junction 71) : {msgData = zeros(0,1);
        | res = false;}
    (junction 71) -> (junction 76) [order 1] : SLOWDOWN
    (junction 76) -> (junction 77) : {msgData = SLOWDOWN.data;
        | TRASH.data = SLOWDOWN.data;
        | forward(SLOWDOWN,TRASH);}
    (junction 77) -> (junction 71) : {res = true;}
    (junction 71) -> (junction 81) [order 2]
  state Forward [parallel]
    on BRAKE:
    SLOWDOWN.data = BRAKE.data;
    forward(BRAKE,SLOWDOWN);
    on PEDES:
    SLOWDOWN.data = [0; A_MAX];
    forward(PEDES,SLOWDOWN);
    settings: executionOrder=2
  state Core [parallel]
    settings: executionOrder=1
    state Straight
      state Stop
      state SlowDown
        en:
        vtarget = msgData(1);
        brake = msgData(2);
        du:
        d = D(:,this);
        accelerate(this, brake*d*(-1));
      state AccToFixedRate
        state Acc
          du:
          d = D(:,this);
          accelerate(this, A_MAX*d);
        state FixRate
          du:
          fixedRate(this);
        Acc -> FixRate : [reachTargetRate(this,vtarget)]
            | {setTargetRate(this,vtarget);}
        (default) -> FixRate [order 1] : [norm(V(:,this)) >= vtarget]
        FixRate -> Acc : [receiveGas && msgData(1) > vtarget]
            | {vtarget = msgData(1);}
        (default) -> Acc [order 2]
      (default) -> Stop [order 1] : [norm(V(:,this)) == 0]
      Stop -> Stop [order 2] : [needSlowDown]
      SlowDown -> SlowDown [order 2] : [needSlowDown && ...
          | norm(V(:,this)) >= msgData(1)]
      (junction 28) -> Stop [order 1] : [vtarget == 0]
      SlowDown -> (junction 28) [order 1] : [reachTargetRate(this,vtarget)]
          | {setTargetRate(this,vtarget);}
      (junction 28) -> FixRate [order 2]
      Stop -> AccToFixedRate [order 1] : [receiveGas]
          | {vtarget = msgData(1);}
      SlowDown -> AccToFixedRate [order 3] : [receiveGas]
          | {vtarget = msgData(1);}
      AccToFixedRate -> SlowDown : [needSlowDown && ...
          | norm(V(:,this)) >= msgData(1)]
      (default) -> AccToFixedRate [order 2]
    state Turn
      en:
      radius = msgData(1);
      state Normal
        du:
        dtheta = norm(V(:,this)) * dt / radius;
        turnDrive(this,radius,dtheta);
      state Halt
        entry: V(:,this) = 0*V(:,this);
      (default) -> Normal
      Halt -> Normal : [receiveGas]{
          | V(:,this) = ...
          | D(:,this)*V_TURN;}
      Normal -> Halt : [needSlowDown]
    (default) -> Straight
    Straight -> Turn : [receiveTurn]
    Turn -> Turn [order 2] : [receiveTurn]
    Turn -> Straight [order 1] : [receiveBack]
  data: res function_output; res function_output; self function_input; r function_input; theta function_input; res function_output; self function_input; a function_input; self function_input; res function_output; self function_input; target function_input; self function_input uint8 size=1; res function_output boolean size=1; target function_input; V_TURN constant double size=1 =1.0; X data_store_memory; V data_store_memory; dt parameter; this local uint8 size=1 =uint8(2); A_MAX constant double =2.5; d local; vtarget local double =2.5; GAS input; WORLD_SIZE parameter; D data_store_memory; TURN input; radius local; dtheta local; BACK input; brake local =2.5; TRASH local; msgData local size=[5 1]; PEDES input; BRAKE input; SLOWDOWN local double
  function turnDrive(self,r,theta):
    | function turnDrive(self, r, theta)
    | 
    | x = X(:,self);
    | v = V(:,self);
    | d = D(:,self);
    | 
    | rot1 = [cos(theta) sin(theta); -sin(theta) cos(theta)];
    | rot2 = [cos(theta/2) sin(theta/2); -sin(theta/2) cos(theta/2)];
    | 
    | v = rot1 * v;
    | d = rot2 * d;
    | 
    | dx = r * sin(theta/2) * d;
    | x = x + dx;
    | 
    | X(:,self) = x;
    | V(:,self) = v;
    | D(:,self) = d;
  function accelerate(self, a):
    | function accelerate(self, a)
    |  
    | x = X(:,self);
    | v = V(:,self);
    | 
    | x = x + v * dt + 0.5 * a * dt * dt;
    | v = v + a * dt;
    | 
    | % a rounded world
    | if x(1) > WORLD_SIZE
    |     x(1) = -WORLD_SIZE;
    | elseif x(1) < -WORLD_SIZE
    |     x(1) = WORLD_SIZE;
    | elseif x(2) > WORLD_SIZE
    |     x(2) = -WORLD_SIZE;
    | elseif x(2) < -WORLD_SIZE
    |     x(2) = WORLD_SIZE;
    | end
    | 
    | X(:,self) = x;
    | V(:,self) = v;
  function fixedRate(self):
    | function fixedRate(self)
    | 
    | x = X(:,self);
    | v = V(:,self);
    | 
    | % update new position
    | x = x + v * dt;
    | 
    | % a rounded world
    | if x(1) > WORLD_SIZE
    |     x(1) = -WORLD_SIZE;
    | elseif x(1) < -WORLD_SIZE
    |     x(1) = WORLD_SIZE;
    | elseif x(2) > WORLD_SIZE
    |     x(2) = -WORLD_SIZE;
    | elseif x(2) < -WORLD_SIZE
    |     x(2) = WORLD_SIZE;
    | end
    | 
    | X(:,self) = x;
  function setTargetRate(self,target):
    | function setTargetRate(self,target)
    | 
    | d = D(:,self);
    | V(:,self) = d * target;
  function res = reachTargetRate(self, target):
    | function res = reachTargetRate(self, target)
    | 
    | res = abs(target - norm(V(:,self))) < 0.125;
